simulink model "Q3_b1_15"  (R2015a)
settings: Solver=ode45  StartTime=0.0  StopTime=10.0  RelTol=1e-3
undefined symbols (not defined in the file or in its folder): K2
libraries: cstblocks x7
settings Model: Creator=yarde_000  LastModifiedBy=yarde_000

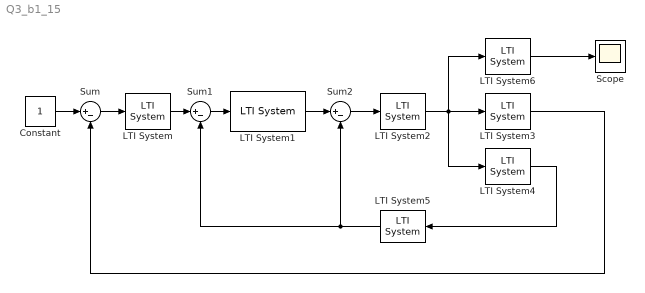
== system Q3_b1_15 ==
  Constant : Constant
  LTI System : cstblocks/LTI System  sys=K3  IC=[]
  LTI System1 : cstblocks/LTI System  sys=K2*tf(1,[1 0])  IC=[]
  LTI System2 : cstblocks/LTI System  sys=K1  IC=[]
  LTI System3 : cstblocks/LTI System  sys=Pa_m  IC=[]
  LTI System4 : cstblocks/LTI System  sys=Pq  IC=[]
  LTI System5 : cstblocks/LTI System  sys=H  IC=[]
  LTI System6 : cstblocks/LTI System  sys=Pa  IC=[]
  Scope : Scope
      settings: YMin=-0.76371  YMax=1.34677  SaveName=Sim_Out
  Sum : Sum  Inputs=|+-
  Sum1 : Sum  Inputs=|+-
  Sum2 : Sum  Inputs=|+-
  wires:
  Sum/1 -> LTI System/1
  Constant/1 -> Sum/1
  LTI System/1 -> Sum1/1
  Sum1/1 -> LTI System1/1
  LTI System1/1 -> Sum2/1
  Sum2/1 -> LTI System2/1
  LTI System2/1 -> LTI System6/1, LTI System3/1, LTI System4/1
  LTI System4/1 -> LTI System5/1
  LTI System6/1 -> Scope/1
  LTI System3/1 -> Sum/2
  LTI System5/1 -> Sum1/2, Sum2/2
